simulink model "PID_Controller_DC_Motor"  (R2020b)
settings: Solver=VariableStepAuto  StartTime=0.0  StopTime=10.0  RelTol=1e-3
settings Model: Creator=SWARUP  LastModifiedBy=SWARUP

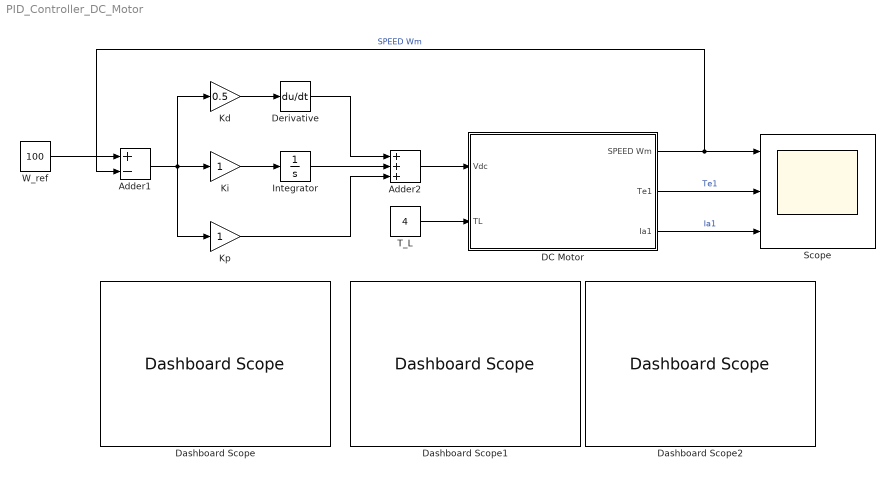
== system PID_Controller_DC_Motor ==
  Adder1 : Sum  Inputs=+-
  Adder2 : Sum  Inputs=+++
  DC Motor : Subsystem
  Dashboard Scope : DashboardScope
  Dashboard Scope1 : DashboardScope
  Dashboard Scope2 : DashboardScope
  "Derivative " : Derivative
  "Integrator " : Integrator
  Kd : Gain  Gain=0.5
  Ki : Gain
  Kp : Gain
  "Scope " : Scope  NumInputPorts=3
  T_L : Constant  Value=4
  W_ref : Constant  Value=100
  wires:
  "Derivative "/1 -> Adder2/1
  "Integrator "/1 -> Adder2/2
  Kp/1 -> Adder2/3
  Ki/1 -> "Integrator "/1
  Kd/1 -> "Derivative "/1
  Adder2/1 -> DC Motor/1(Vdc)
  T_L/1 -> DC Motor/2(TL)
  DC Motor/1(SPEED Wm) -> "Scope "/1, Adder1/2  "SPEED Wm"
  DC Motor/2(Te1) -> "Scope "/2  "Te1"
  DC Motor/3(Ia1) -> "Scope "/3  "Ia1"
  Adder1/1 -> Kd/1, Kp/1, Ki/1
  W_ref/1 -> Adder1/1

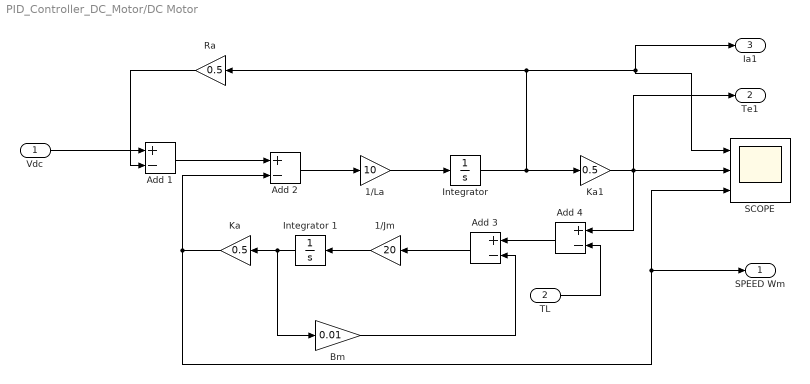
== system PID_Controller_DC_Motor/DC Motor ==
  Vdc : Inport
  TL : Inport  Port=2
  1/Jm : Gain  Gain=20
  1/La : Gain  Gain=10
  Add {1..4} (4 alike) : Sum  Inputs=+-
  Bm : Gain  Gain=0.01
  "Integrator " : Integrator
  Integrator 1 : Integrator
  Ka : Gain  Gain=0.5
  Ka1 : Gain  Gain=0.5
  Ra : Gain  Gain=0.5
  SCOPE : Scope  NumInputPorts=3
  SPEED Wm : Outport
  Te1 : Outport  Port=2
  Ia1 : Outport  Port=3
  wires:
  "Integrator "/1 -> Ia1/1, SCOPE/1, Ra/1, Ka1/1
  Ra/1 -> Add 1/2
  Ka1/1 -> Te1/1, SCOPE/2, Add 4/1
  Add 1/1 -> Add 2/1
  Ka/1 -> Add 2/2, SPEED Wm/1, SCOPE/3
  TL/1 -> Add 4/2
  Bm/1 -> Add 3/2
  Add 3/1 -> 1/Jm/1
  Integrator 1/1 -> Bm/1, Ka/1
  1/La/1 -> "Integrator "/1
  Add 4/1 -> Add 3/1
  1/Jm/1 -> Integrator 1/1
  Vdc/1 -> Add 1/1
  Add 2/1 -> 1/La/1
